simulink library "crop_cost"  (R2025b)
settings: Solver=VariableStepAuto  StartTime=0.0  StopTime=10.0  RelTol=1e-3
settings Model: Creator=ciepm  LastModifiedBy=charlielenk

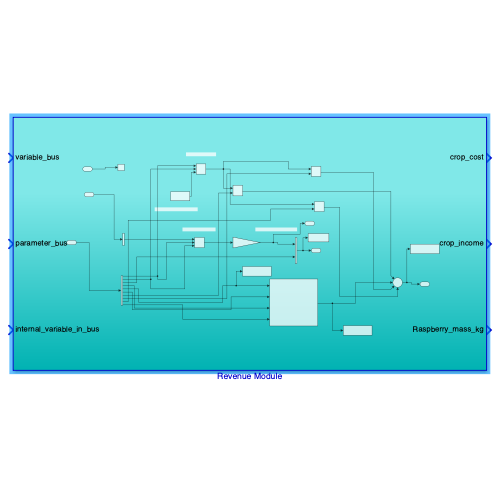
[thumbnail: Simulink's stored preview of the top-level diagram]
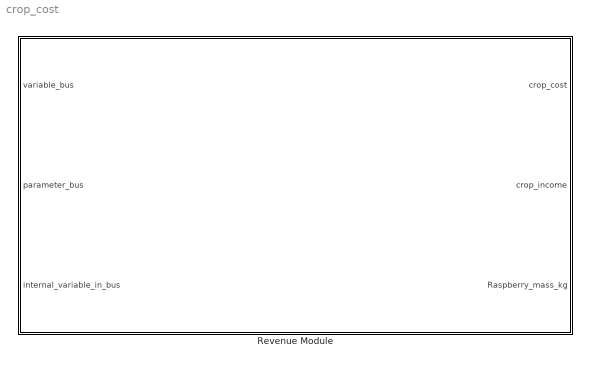
== system crop_cost ==
  Revenue Module : Subsystem

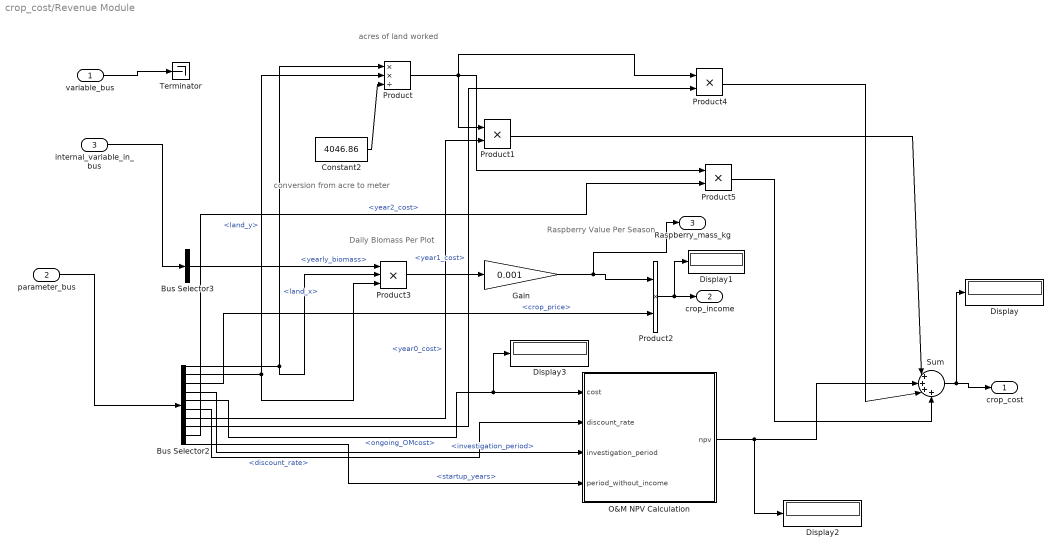
== system crop_cost/Revenue Module ==
  note: Daily Biomass Per Plot
  note: Raspberry Value Per Season
  note: acres of land worked
  note: conversion from acre to meter
  variable_bus : Inport
  parameter_bus : Inport  Port=2
  internal_variable_in_bus : Inport  Port=3
  Bus Selector2 : BusSelector  OutputSignals=land_x,land_y,crop_price,investigation_period,ongoing_OMcost,discount_rate,year0_cost,year1_cost,year2_cost,startup_years
  Bus Selector3 : BusSelector  OutputSignals=yearly_biomass
  Constant2 : Constant  Value=4046.86
  Display{,1..3} (4 alike) : Display
  Gain : Gain  Gain=0.001
  O&M NPV Calculation : MATLAB Function  TreatAsAtomicUnit=on
  Product : Product  Inputs=**/
  Product{1..2,4..5} (4 alike) : Product
  Product3 : Product  Inputs=3
  Sum : Sum  Inputs=|++++
  Terminator : Terminator
  crop_cost : Outport
  crop_income : Outport  Port=2
  Raspberry_mass_kg : Outport  Port=3
  wires:
  Bus Selector2/10 -> O&M NPV Calculation/4(period_without_income)  "<startup_years>"
  Bus Selector2/9 -> Product5/2  "<year2_cost>"
  Bus Selector2/8 -> Product4/2  "<year1_cost>"
  Bus Selector2/7 -> Product1/2  "<year0_cost>"
  variable_bus/1 -> Terminator/1
  Product5/1 -> Sum/4
  Product4/1 -> Sum/3
  Product1/1 -> Sum/1
  Sum/1 -> crop_cost/1, Display/1
  O&M NPV Calculation/1(npv) -> Display2/1, Sum/2
  Bus Selector2/6 -> O&M NPV Calculation/2(discount_rate)  "<discount_rate>"
  Bus Selector2/5 -> Display3/1, O&M NPV Calculation/1(cost)  "<ongoing_OMcost>"
  Bus Selector2/4 -> O&M NPV Calculation/3(investigation_period)  "<investigation_period>"
  Product/1 -> Product4/1, Product1/1, Product5/1
  Constant2/1 -> Product/3
  Product2/1 -> crop_income/1, Display1/1
  Bus Selector3/1 -> Product3/1  "<yearly_biomass>"
  Bus Selector2/1 -> Product/1, Product3/2  "<land_x>"
  Bus Selector2/2 -> Product/2, Product3/3  "<land_y>"
  Bus Selector2/3 -> Product2/2  "<crop_price>"
  Gain/1 -> Product2/1, Raspberry_mass_kg/1
  Product3/1 -> Gain/1
  parameter_bus/1 -> Bus Selector2/1
  internal_variable_in_bus/1 -> Bus Selector3/1

== matlab function crop_cost/Revenue Module/O&M NPV Calculation ==
  data: cost input; npv output; discount_rate input; investigation_period input; period_without_income input
function npv = calc_discounted_cash_flow(cost, discount_rate, investigation_period,period_without_income)
    exponent_value = period_without_income:investigation_period-1;
    npv = sum(cost ./ (1 + discount_rate).^exponent_value);
end
